simulink model "Android_Sensors_UDP"  (R2023a)
settings: Solver=FixedStepAuto  StartTime=0.0  StopTime=10.0  RelTol=1e-3
model workspace (MAT data in the model file):
  IP_Addr = '255.255.255.255'
libraries: androiduilib x10, androidsensorlib x9, simulink x1, androidcommunicationlib x1
settings Model: Creator=The MathWorks, Inc.  LastModifiedBy=muham
settings SolverCC: AlgebraicLoopSolver=TrustRegion
settings OptimizationCC: EnhancedBackFolding=on  PassReuseOutputArgsThreshold=0  MaxStackSize=64  OptimizeBlockOrder=speed  DifferentSizesBufferReuse=on  OptimizationCustomize=off
settings DebuggingCC: ParameterTunabilityLossMsg=error  UnconnectedInputMsg=warning  UnconnectedOutputMsg=warning  UnconnectedLineMsg=warning  ArithmeticOperatorsInVariantConditions=warning
settings HardwareCC: ProdBitPerPointer=32  ProdBitPerSizeT=32  ProdBitPerPtrDiffT=32  ProdLargestAtomicInteger=Long  ProdLargestAtomicFloat=Double  ProdWordSize=32  ProdHWDeviceType=ARM Compatible->ARM Cortex  UseEmbeddedCoderFeatures=off  UseSimulinkCoderFeatures=off
settings ModelReferenceCC: EnableRefExpFcnMdlSchedulingChecks=on
settings SFSimCC: MATLABDynamicMemAlloc=off  CustomCodeUndefinedFunction=UseInterfaceOnly
settings RTWCC: Description=Embedded Coder  SystemTargetFile=ert.tlc  HardwareBoard=Android Device  TLCOptions="-aInlineSetEventsForThisBaseRateFcn=TLC_FALSE -aSuppressMultiTaskScheduler=TLC_FALSE  -aRateBasedStepFcn=0"  TemplateMakefile=ert_default_tmf  GenerateReport=on  RTWVerbose=off  Toolchain=Android SDK/NDK Tools  LaunchReport=on  DLArmComputeVersion=19.05
settings CodeAppCC: ForceParamTrailComments=on  OperatorAnnotations=on
settings ERTTargetCC: ERTCustomFileBanners=off  SupportContinuousTime=on  SupportNonInlinedSFcns=on  RemoveResetFunc=off  ModelStepFunctionPrototypeControlCompliant=off

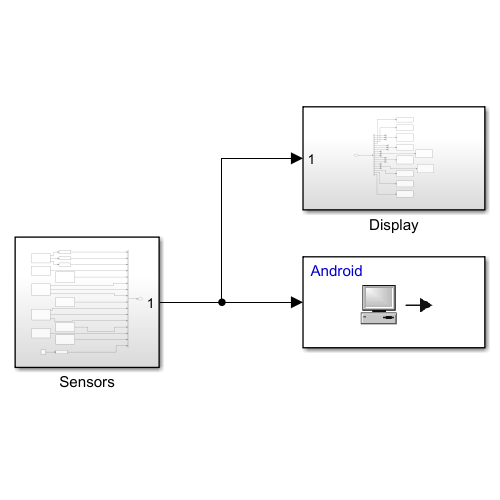
[thumbnail: Simulink's stored preview of the top-level diagram]
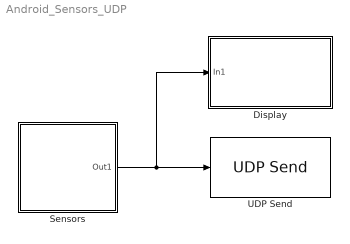
== system Android_Sensors_UDP ==
  Display : Subsystem
  Sensors : Subsystem
  UDP Send : androidcommunicationlib/UDP Send  remoteURL='255.255.255.255'  remotePort=25000  localURL='0.0.0.0'  localPortSource=Automatically determine  localPort=-1  sampletime=-1  blockPlatform=Android  separateLengthPort=0
  wires:
  Sensors/1(Out1) -> UDP Send/1, Display/1(In1)

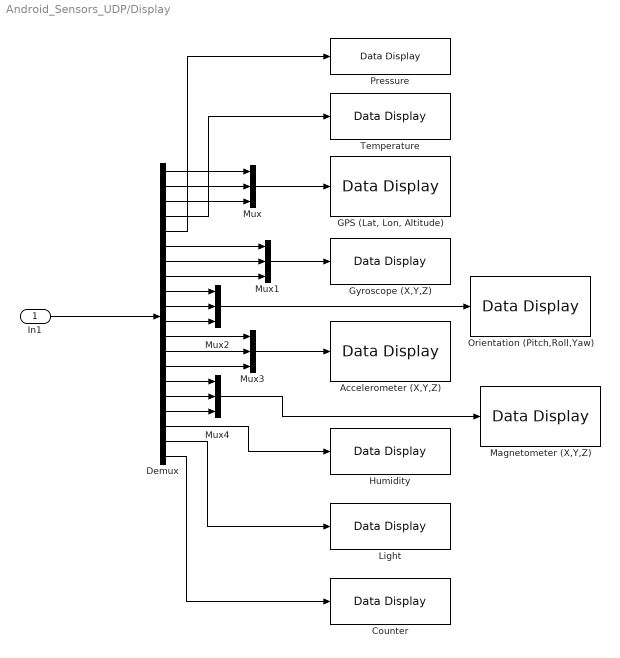
== system Android_Sensors_UDP/Display ==
  In1 : Inport
  Accelerometer (X,Y,Z) : androiduilib/Data Display  DataDisplayId=Android_Sensors_UDP/Display/Data_Display  Format=Float  Precision=6  SimulateUsing=Code generation  blockPlatform=Android
  Counter : androiduilib/Data Display  DataDisplayId=Android_Sensors_UDP/Display/Data_Display  Format=Float  Precision=6  SimulateUsing=Code generation  blockPlatform=Android
  Demux : Demux  Outputs=20
  "GPS (Lat, Lon, Altitude)" : androiduilib/Data Display  DataDisplayId=Android_Sensors_UDP/Display/Data_Display  Format=Float  Precision=6  SimulateUsing=Code generation  blockPlatform=Android
  Gyroscope (X,Y,Z) : androiduilib/Data Display  DataDisplayId=Android_Sensors_UDP/Display/Data_Display  Format=Float  Precision=6  SimulateUsing=Code generation  blockPlatform=Android
  Humidity : androiduilib/Data Display  DataDisplayId=Android_Sensors_UDP/Display/Data_Display  Format=Float  Precision=6  SimulateUsing=Code generation  blockPlatform=Android
  Light : androiduilib/Data Display  DataDisplayId=Android_Sensors_UDP/Display/Data_Display  Format=Float  Precision=6  SimulateUsing=Code generation  blockPlatform=Android
  Magnetometer (X,Y,Z) : androiduilib/Data Display  DataDisplayId=Android_Sensors_UDP/Display/Data_Display  Format=Float  Precision=6  SimulateUsing=Code generation  blockPlatform=Android
  Mux{,1..4} (5 alike) : Mux  Inputs=3
  Orientation (Pitch,Roll,Yaw) : androiduilib/Data Display  DataDisplayId=Android_Sensors_UDP/Display/Data_Display  Format=Float  Precision=6  SimulateUsing=Code generation  blockPlatform=Android
  Pressure : androiduilib/Data Display  DataDisplayId=Android_Sensors_UDP/Display/Data_Display  Format=Float  Precision=6  SimulateUsing=Code generation  blockPlatform=Android
  Temperature : androiduilib/Data Display  DataDisplayId=Android_Sensors_UDP/Display/Data_Display  Format=Float  Precision=6  SimulateUsing=Code generation  blockPlatform=Android
  wires:
  In1/1 -> Demux/1
  Demux/1 -> Mux/1
  Demux/2 -> Mux/2
  Demux/3 -> Mux/3
  Mux/1 -> "GPS (Lat, Lon, Altitude)"/1
  Demux/4 -> Temperature/1
  Demux/5 -> Pressure/1
  Demux/8 -> Mux1/3
  Demux/6 -> Mux1/1
  Mux1/1 -> Gyroscope (X,Y,Z)/1
  Demux/7 -> Mux1/2
  Demux/11 -> Mux2/3
  Demux/9 -> Mux2/1
  Mux2/1 -> Orientation (Pitch,Roll,Yaw)/1
  Demux/10 -> Mux2/2
  Demux/14 -> Mux3/3
  Demux/12 -> Mux3/1
  Mux3/1 -> Accelerometer (X,Y,Z)/1
  Demux/13 -> Mux3/2
  Demux/17 -> Mux4/3
  Demux/15 -> Mux4/1
  Demux/16 -> Mux4/2
  Mux4/1 -> Magnetometer (X,Y,Z)/1
  Demux/18 -> Humidity/1
  Demux/19 -> Light/1
  Demux/20 -> Counter/1

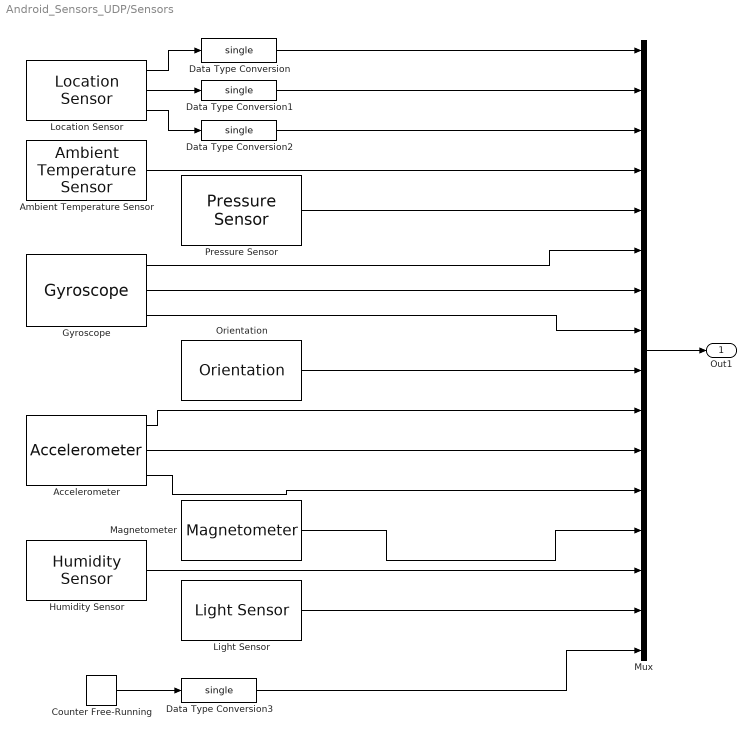
== system Android_Sensors_UDP/Sensors ==
  Accelerometer : androidsensorlib/Accelerometer  OutputVector=off  SampleTime=0.01  BlockPlatform=Android
  Ambient Temperature Sensor : androidsensorlib/Ambient Temperature Sensor  SampleTime=0.01  BlockPlatform=Android
  Counter Free-Running : simulink/Sources/Counter Free-Running  NumBits=24  tsamp=0.01
  Data Type Conversion{,1..3} (4 alike) : DataTypeConversion  OutDataTypeStr=single  SaturateOnIntegerOverflow=off  RndMeth=Floor
  Gyroscope : androidsensorlib/Gyroscope  OutputVector=off  SampleTime=0.01  BlockPlatform=Android
  Humidity Sensor : androidsensorlib/Humidity Sensor  SampleTime=0.01  BlockPlatform=Android
  Light Sensor : androidsensorlib/Light Sensor  SampleTime=0.01  BlockPlatform=Android
  Location Sensor : androidsensorlib/Location Sensor  OutputVector=off  SampleTime=0.01  BlockPlatform=Android
  Magnetometer : androidsensorlib/Magnetometer  SampleTime=0.01
  Mux : Mux  Inputs=16
  Orientation : androidsensorlib/Orientation  SampleTime=0.01
  Pressure Sensor : androidsensorlib/Pressure Sensor  BlockPlatform=Android  SampleTime=0.01
  Out1 : Outport
  wires:
  Gyroscope/3 -> Mux/8
  Data Type Conversion/1 -> Mux/1
  Location Sensor/3 -> Data Type Conversion2/1
  Location Sensor/2 -> Data Type Conversion1/1
  Data Type Conversion1/1 -> Mux/2
  Accelerometer/3 -> Mux/12
  Accelerometer/1 -> Mux/10
  Location Sensor/1 -> Data Type Conversion/1
  Pressure Sensor/1 -> Mux/5
  Counter Free-Running/1 -> Data Type Conversion3/1
  Gyroscope/1 -> Mux/6
  Accelerometer/2 -> Mux/11
  Humidity Sensor/1 -> Mux/14
  Mux/1 -> Out1/1
  Data Type Conversion3/1 -> Mux/16
  Ambient Temperature Sensor/1 -> Mux/4
  Data Type Conversion2/1 -> Mux/3
  Magnetometer/1 -> Mux/13
  Light Sensor/1 -> Mux/15
  Orientation/1 -> Mux/9
  Gyroscope/2 -> Mux/7
